simulink model "servo_motor_model"  (R2024a)
settings: Solver=VariableStepAuto  StartTime=0.0  StopTime=10.0  RelTol=1e-3
settings Model: Creator=s14  LastModifiedBy=s14

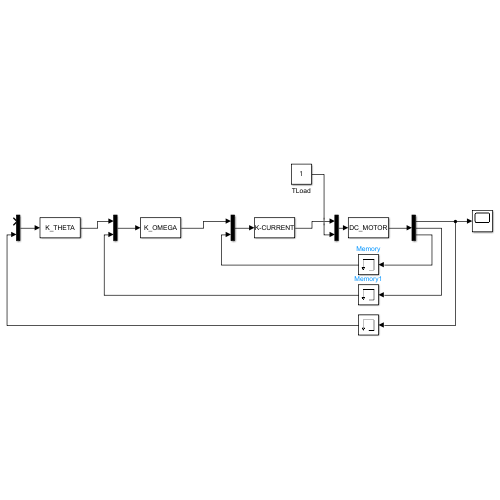
[thumbnail: Simulink's stored preview of the top-level diagram]
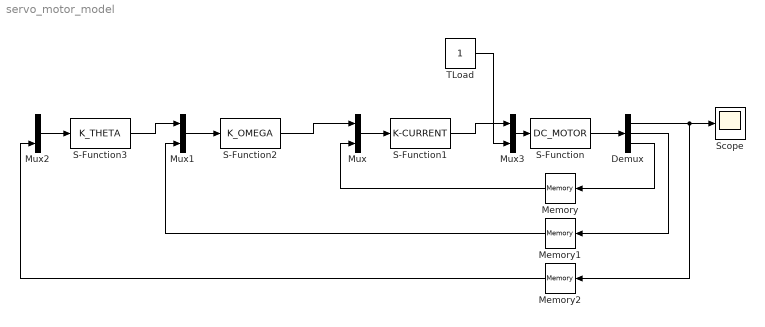
== system servo_motor_model ==
  Demux : Demux  Outputs=3
  Memory : Memory
  Memory1 : Memory
  Memory2 : Memory
  Mux{,1..3} (4 alike) : Mux  Inputs=2
  S-Function : S-Function  FunctionName=DC_MOTOR  SFunctionDeploymentMode=off  EnableBusSupport=off
  S-Function1 : S-Function  FunctionName=K-CURRENT  SFunctionDeploymentMode=off  EnableBusSupport=off
  S-Function2 : S-Function  FunctionName=K_OMEGA  SFunctionDeploymentMode=off  EnableBusSupport=off
  S-Function3 : S-Function  FunctionName=K_THETA  SFunctionDeploymentMode=off  EnableBusSupport=off
  Scope : Scope
  TLoad : Constant
  wires:
  S-Function/1 -> Demux/1
  Mux/1 -> S-Function1/1
  S-Function2/1 -> Mux/1
  Mux1/1 -> S-Function2/1
  S-Function3/1 -> Mux1/1
  Mux2/1 -> S-Function3/1
  Mux3/1 -> S-Function/1
  S-Function1/1 -> Mux3/1
  TLoad/1 -> Mux3/2
  Demux/3 -> Memory/1
  Memory/1 -> Mux/2
  Demux/2 -> Memory1/1
  Memory1/1 -> Mux1/2
  Demux/1 -> Memory2/1, Scope/1
  Memory2/1 -> Mux2/2
